simulink library "xpcnilib"  (Simulink 6.0)
settings: Solver=ode45  SolverMode=SingleTasking  StartTime=0.0  StopTime=10.0  RelTol=1e-3
undefined symbols (not defined in the file or in its folder): madnipcie, mctrnipcie, mctrnipciecap, mdacbisa, mdanipci670x, mdanipci671x, mdanipcie, mdionipci6527, mdionipcie, mencnipci660x, misa8255, mnigpib, mnipci660x, mpci8255
libraries: xpcmeasurementcomputinglib x6
(part 2 of 3)

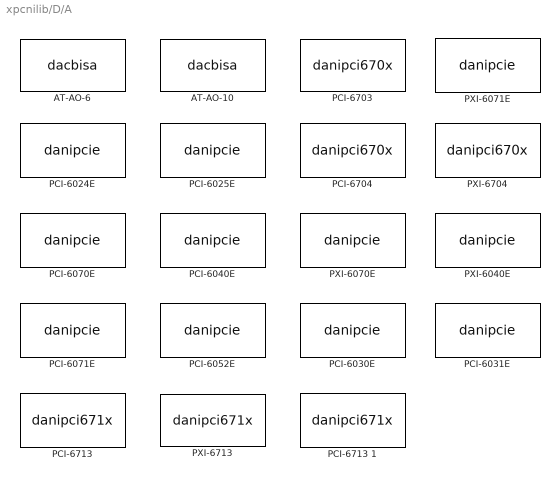
== system xpcnilib/D/A ==
  "AT-AO-10 " : S-Function  InitFcn=mdacbisa(1);  FunctionName=dacbisa  Parameters=channel, range, reset, initValue, sampletime, baseaddress, boardType  mask(dacbisa){channel=[1], range=[-10], reset=[1], initValue=[0], sampletime=0.001, baseaddress=0x300}
      mask prompts: channel "Channel vector:"; range "Range vector:"; reset "Reset vector:"; initValue "Initial value vector:"; sampletime "Sample time:"; baseaddress "Base address (i.e. 0xd000):"
      mask help:
      | AT-AO-10
      | National Instr.
      | Analog Output
      mask init:
      | baseaddress=hex2dec(baseaddress(3:end));
      | boardType=12;
      | [reset, initValue] = mdacbisa(2, channel, range, reset, initValue, baseaddress, boardType);
      mask Help: helpview(fullfile(docroot, 'mapfiles', 'xpc.map'), 'NationalInstruments_AT-AO-10_DA')
      mask Display: disp('AT-AO-10\nNational Instr.\nAnalog Output');port_label('input',1,'1');
  "AT-AO-6 " : S-Function  InitFcn=mdacbisa(1);  FunctionName=dacbisa  Parameters=channel, range, reset, initValue, sampletime, baseaddress, boardType  mask(dacbisa){channel=[1], range=[-10], reset=[1], initValue=[0], sampletime=0.001, baseaddress=0x300}
      mask prompts: channel "Channel vector:"; range "Range vector:"; reset "Reset vector:"; initValue "Initial value vector:"; sampletime "Sample time:"; baseaddress "Base address (i.e. 0xd000):"
      mask help:
      | AT-AO-6
      | National Instr.
      | Analog Output
      mask init:
      | baseaddress=hex2dec(baseaddress(3:end));
      | boardType=11;
      | [reset, initValue] = mdacbisa(2, channel, range, reset, initValue, baseaddress, boardType);
      mask Help: helpview(fullfile(docroot, 'mapfiles', 'xpc.map'), 'NationalInstruments_AT-AO-6_DA')
      mask Display: disp('AT-AO-6\nNational Instr.\nAnalog Output');port_label('input',1,'1');
  "PCI-6024E " : S-Function  InitFcn=mdanipcie(1);  FunctionName=danipcie  Parameters="channel, range, reset, initValue, sampletime, slot,  boardType"  mask(danipcie){channel=[1], reset=[1], initValue=[0], sampletime=0.001, slot=-1}
      mask prompts: channel "Channel vector:"; reset "Reset vector:"; initValue "Initial value vector:"; sampletime "Sample time:"; slot "PCI slot (-1: autosearch):"
      mask help:
      | PCI-6024E
      | National Instruments
      | Analog Output
      mask init:
      | boardType=2;
      | range=[];
      | [range,reset,initValue]=mdanipcie(2,channel, range, reset, initValue, slot, boardType);
      mask Help: helpview(fullfile(docroot, 'mapfiles', 'xpc.map'), 'NationalInstruments_PCI-6024E_DA')
      mask Display: disp('PCI-6024E\nNational Instr.\nAnalog Output');port_label('input',1,'1');
  "PCI-6025E " : S-Function  InitFcn=mdanipcie(1);  FunctionName=danipcie  Parameters="channel, range, reset, initValue, sampletime, slot,  boardType"  mask(danipcie){channel=[1], reset=[1], initValue=[0], sampletime=0.001, slot=-1}
      mask prompts: channel "Channel vector:"; reset "Reset vector:"; initValue "Initial value vector:"; sampletime "Sample time:"; slot "PCI slot (-1: autosearch):"
      mask help:
      | PCI-6025E
      | National Instruments
      | Analog Output
      mask init:
      | boardType=3;
      | range=[];
      | [range, reset, initValue]=mdanipcie(2,channel, range, reset, initValue, slot, boardType);
      mask Help: helpview(fullfile(docroot, 'mapfiles', 'xpc.map'), 'NationalInstruments_PCI-6025E_DA')
      mask Display: disp('PCI-6025E\nNational Instr.\nAnalog Output');port_label('input',1,'1');
  "PCI-6030E " : S-Function  InitFcn=mdanipcie(1);  FunctionName=danipcie  Parameters="channel, range, reset, initValue, sampletime, slot,  boardType"  mask(danipcie){channel=[1], range=[-10], reset=[1], initValue=[0], sampletime=0.001, slot=-1}
      mask prompts: channel "Channel vector:"; range "Range vector:"; reset "Reset vector:"; initValue "Initial value vector:"; sampletime "Sample time:"; slot "PCI slot (-1: autosearch):"
      mask help:
      | PCI-6030E
      | National Instruments
      | Analog Output
      mask init:
      | boardType=10;
      | [range,reset,initValue]=mdanipcie(2,channel, range, reset, initValue, slot, boardType);
      mask Help: helpview(fullfile(docroot, 'mapfiles', 'xpc.map'), 'NationalInstruments_PCI-MIO-16XE-10_DA')
      mask Display: disp('PCI-6030E\nNational Instr.\nAnalog Output');port_label('input',1,'1');
  "PCI-6031E " : S-Function  InitFcn=mdanipcie(1);  FunctionName=danipcie  Parameters="channel, range, reset, initValue, sampletime, slot,  boardType"  mask(danipcie){channel=[1], range=[-10], reset=[1], initValue=[0], sampletime=0.001, slot=-1}
      mask prompts: channel "Channel vector:"; range "Range vector:"; reset "Reset vector:"; initValue "Initial value vector:"; sampletime "Sample time:"; slot "PCI slot (-1: autosearch):"
      mask help:
      | PCI-6031E
      | National Instruments
      | Analog Output
      mask init:
      | boardType=11;
      | [range,reset,initValue]=mdanipcie(2,channel, range, reset, initValue, slot, boardType);
      mask Help: helpview(fullfile(docroot, 'mapfiles', 'xpc.map'), 'NationalInstruments_PCI-6031E_DA')
      mask Display: disp('PCI-6031E\nNational Instr.\nAnalog Output');port_label('input',1,'1');
  "PCI-6040E " : S-Function  InitFcn=mdanipcie(1);  FunctionName=danipcie  Parameters="channel, range, reset, initValue, sampletime, slot,  boardType"  mask(danipcie){channel=[1], range=[-10], reset=[1], initValue=[0], sampletime=0.001, slot=-1}
      mask prompts: channel "Channel vector:"; range "Range vector:"; reset "Reset vector:"; initValue "Initial value vector:"; sampletime "Sample time:"; slot "PCI slot (-1: autosearch):"
      mask help:
      | PCI-6040E
      | National Instruments
      | Analog Output
      mask init:
      | boardType=5;
      | [range,reset,initValue]=mdanipcie(2,channel, range, reset, initValue, slot, boardType);
      mask Help: helpview(fullfile(docroot, 'mapfiles', 'xpc.map'), 'NationalInstruments_PCI-MIO-16E-4_DA')
      mask Display: disp('PCI-6040E\nNational Instr.\nAnalog Output');port_label('input',1,'1');
  "PCI-6052E " : S-Function  InitFcn=mdanipcie(1);  FunctionName=danipcie  Parameters="channel, range, reset, initValue, sampletime, slot,  boardType"  mask(danipcie){channel=[1], range=[-10], reset=[1], initValue=[0], sampletime=0.001, slot=-1}
      mask prompts: channel "Channel vector:"; range "Range vector:"; reset "Reset vector:"; initValue "Initial value vector:"; sampletime "Sample time:"; slot "PCI slot (-1: autosearch):"
      mask help:
      | PCI-6052E
      | National Instruments
      | Analog Output
      mask init:
      | boardType=9;
      | [range,reset,initValue]=mdanipcie(2,channel, range, reset, initValue, slot, boardType);
      mask Help: helpview(fullfile(docroot, 'mapfiles', 'xpc.map'), 'NationalInstruments_PCI-6052E_DA')
      mask Display: disp('PCI-6052E\nNational Instr.\nAnalog Output');port_label('input',1,'1');
  "PCI-6070E " : S-Function  InitFcn=mdanipcie(1);  FunctionName=danipcie  Parameters="channel, range, reset, initValue, sampletime, slot,  boardType"  mask(danipcie){channel=[1], range=[-10], reset=[1], initValue=[0], sampletime=0.001, slot=-1}
      mask prompts: channel "Channel vector:"; range "Range vector:"; reset "Reset vector:"; initValue "Initial value vector:"; sampletime "Sample time:"; slot "PCI slot (-1: autosearch):"
      mask help:
      | PCI-6070E
      | National Instruments
      | Analog Output
      mask init:
      | boardType=4;
      | [range,reset,initValue]=mdanipcie(2,channel, range, reset, initValue, slot, boardType);
      mask Help: helpview(fullfile(docroot, 'mapfiles', 'xpc.map'), 'NationalInstruments_PCI-MIO-16E-1_DA')
      mask Display: disp('PCI-6070E\nNational Instr.\nAnalog Output');port_label('input',1,'1');
  "PCI-6071E " : S-Function  InitFcn=mdanipcie(1);  FunctionName=danipcie  Parameters="channel, range, reset, initValue, sampletime, slot,  boardType"  mask(danipcie){channel=[1], range=[-10], reset=[1], initValue=[0], sampletime=0.001, slot=-1}
      mask prompts: channel "Channel vector:"; range "Range vector:"; reset "Reset vector:"; initValue "Initial value vector:"; sampletime "Sample time:"; slot "PCI slot (-1: autosearch):"
      mask help:
      | PCI-6071E
      | National Instruments
      | Analog Output
      mask init:
      | boardType=8;
      | [range,reset,initValue]=mdanipcie(2,channel, range, reset, initValue, slot, boardType);
      mask Help: helpview(fullfile(docroot, 'mapfiles', 'xpc.map'), 'NationalInstruments_PCI-6071E_DA')
      mask Display: disp('PCI-6071E\nNational Instr.\nAnalog Output');port_label('input',1,'1');
  "PCI-6703 " : S-Function  InitFcn=mdanipci670x(1);  FunctionName=danipci670x  Parameters=channel, sampletime, pcislot, boardType  mask(danipci6703){channel=[1], sampletime=0.001, pcislot=-1}
      mask prompts: channel "Channel vector:"; sampletime "Sample time:"; pcislot "PCI slot (-1: autosearch):"
      mask help:
      | PCI-6703
      | National Instr.
      | Analog Output
      mask init:
      | boardType=1;
      | [maskdisplay, maskdescription]= mdanipci670x(2, boardType, channel, pcislot);
      | set_param(gcb,'MaskDescription',maskdescription);
      | set_param(gcb,'MaskDisplay',maskdisplay);
      mask Help: helpview(fullfile(docroot, 'mapfiles', 'xpc.map'), 'NationalInstruments_PCI-6703_DA')
      mask Display: disp('PCI-6703\nNational Instr.\nAnalog Output');port_label('input',1,'1');
  "PCI-6704 " : S-Function  InitFcn=mdanipci670x(1);  FunctionName=danipci670x  Parameters=channel, sampletime, pcislot, boardType  mask(danipci6704){channel=[1], sampletime=0.001, pcislot=-1}
      mask prompts: channel "Channel vector:"; sampletime "Sample time:"; pcislot "PCI slot (-1: autosearch):"
      mask help:
      | PCI-6704
      | National Instr.
      | Analog Output
      mask init:
      | boardType=2;
      | [maskdisplay, maskdescription]= mdanipci670x(2, boardType, channel, pcislot);
      | set_param(gcb,'MaskDescription',maskdescription);
      | set_param(gcb,'MaskDisplay',maskdisplay);
      mask Help: helpview(fullfile(docroot, 'mapfiles', 'xpc.map'), 'NationalInstruments_PCI-6704_DA')
      mask Display: disp('PCI-6704\nNational Instr.\nAnalog Output');port_label('input',1,'1');
  "PCI-6713 " : S-Function  InitFcn=mdanipci671x( 1, 1 );  FunctionName=danipci671x  Parameters=channel, sampletime, pcislot, boardType, reset, initval  mask(danipci6713){channel=[1], reset=[0], initval=[0], sampletime=0.001, pcislot=-1}
      mask prompts: channel "Channel vector:"; reset "Reset vector:"; initval "Initial value vector:"; sampletime "Sample time:"; pcislot "PCI slot (-1: autosearch):"
      mask help:
      | PCI-6713
      | National Instr.
      | Analog Output
      mask init:
      | boardType=1;
      | [maskdisplay, maskdescription, reset, initval]= mdanipci671x(2, boardType, channel, reset, initval, pcislot);
      | set_param(gcb,'MaskDescription',maskdescription);
      | set_param(gcb,'MaskDisplay',maskdisplay);
      mask Help: helpview(fullfile(docroot, 'mapfiles', 'xpc.map'), 'NationalInstruments_PCI-6713_DA')
      mask Display: disp('PCI-6713\nNational Instr.\nAnalog Output');port_label('input',1,'1');
  "PCI-6713 1 " : S-Function  InitFcn=mdanipci671x( 1, 1 );  FunctionName=danipci671x  Parameters=channel, sampletime, pcislot, boardType, reset, initval  mask(danipci6711){channel=[1], reset=[0], initval=[0], sampletime=0.001, pcislot=-1}
      mask prompts: channel "Channel vector:"; reset "Reset vector:"; initval "Initial value vector:"; sampletime "Sample time:"; pcislot "PCI slot (-1: autosearch):"
      mask help:
      | PCI-6711
      | National Instr.
      | Analog Output
      mask init:
      | boardType=3;
      | [maskdisplay, maskdescription, reset, initval]= mdanipci671x(2, boardType, channel, reset, initval, pcislot);
      | set_param(gcb,'MaskDescription',maskdescription);
      | set_param(gcb,'MaskDisplay',maskdisplay);
      mask Help: helpview(fullfile(docroot, 'mapfiles', 'xpc.map'), 'NationalInstruments_PCI-6711_DA')
      mask Display: disp('PCI-6711\nNational Instr.\nAnalog Output');port_label('input',1,'1');
  "PXI-6040E " : S-Function  InitFcn=mdanipcie(1);  FunctionName=danipcie  Parameters="channel, range, reset, initValue, sampletime, slot,  boardType"  mask(danipcie){channel=[1], range=[-10], reset=[1], initValue=[0], sampletime=0.001, slot=-1}
      mask prompts: channel "Channel vector:"; range "Range vector:"; reset "Reset vector:"; initValue "Initial value vector:"; sampletime "Sample time:"; slot "PCI slot (-1: autosearch):"
      mask help:
      | PXI-6040E
      | National Instruments
      | Analog Output
      mask init:
      | boardType=7;
      | [range,reset,initValue]=mdanipcie(2,channel, range, reset, initValue, slot, boardType);
      mask Help: helpview(fullfile(docroot, 'mapfiles', 'xpc.map'), 'NationalInstruments_PXI-6040E_DA')
      mask Display: disp('PXI-6040E\nNational Instr.\nAnalog Output');port_label('input',1,'1');
  "PXI-6070E " : S-Function  InitFcn=mdanipcie(1);  FunctionName=danipcie  Parameters="channel, range, reset, initValue, sampletime, slot,  boardType"  mask(danipcie){channel=[1], range=[-10], reset=[1], initValue=[0], sampletime=0.001, slot=-1}
      mask prompts: channel "Channel vector:"; range "Range vector:"; reset "Reset vector:"; initValue "Initial value vector:"; sampletime "Sample time:"; slot "PCI slot (-1: autosearch):"
      mask help:
      | PXI-6070E
      | National Instruments
      | Analog Output
      mask init:
      | boardType=6;
      | [range,reset,initValue]=mdanipcie(2,channel, range, reset, initValue, slot, boardType);
      mask Help: helpview(fullfile(docroot, 'mapfiles', 'xpc.map'), 'NationalInstruments_PXI-6070E_DA')
      mask Display: disp('PXI-6070E\nNational Instr.\nAnalog Output');port_label('input',1,'1');
  "PXI-6071E " : S-Function  InitFcn=mdanipcie(1);  FunctionName=danipcie  Parameters="channel, range, reset, initValue, sampletime, slot,  boardType"  mask(danipcie){channel=[1], range=[-10], reset=[1], initValue=[0], sampletime=0.001, slot=-1}
      mask prompts: channel "Channel vector:"; range "Range vector:"; reset "Reset vector:"; initValue "Initial value vector:"; sampletime "Sample time:"; slot "PCI slot (-1: autosearch):"
      mask help:
      | PXI-6071E
      | National Instruments
      | Analog Output
      mask init:
      | boardType=12;
      | [range,reset,initValue]=mdanipcie(2,channel, range, reset, initValue, slot, boardType);
      mask Help: helpview(fullfile(docroot, 'mapfiles', 'xpc.map'), 'NationalInstruments_PXI-6071E_DA')
      mask Display: disp('PXI-6071E\nNational Instr.\nAnalog Output');port_label('input',1,'1');
  "PXI-6704 " : S-Function  InitFcn=mdanipci670x(1);  FunctionName=danipci670x  Parameters=channel, sampletime, pcislot, boardType  mask(danipxi6704){channel=[1], sampletime=0.001, pcislot=-1}
      mask prompts: channel "Channel vector:"; sampletime "Sample time:"; pcislot "PCI slot (-1: autosearch):"
      mask help:
      | PXI-6704
      | National Instr.
      | Analog Output
      mask init:
      | boardType=3;
      | [maskdisplay, maskdescription]= mdanipci670x(2, boardType, channel, pcislot);
      | set_param(gcb,'MaskDescription',maskdescription);
      | set_param(gcb,'MaskDisplay',maskdisplay);
      mask Help: helpview(fullfile(docroot, 'mapfiles', 'xpc.map'), 'NationalInstruments_PCI-6704_DA')
      mask Display: disp('PXI-6704\nNational Instr.\nAnalog Output');port_label('input',1,'1');
  "PXI-6713 " : S-Function  InitFcn=mdanipci671x( 1, 2 );  FunctionName=danipci671x  Parameters=channel, sampletime, pcislot, boardType, reset, initval  mask(danipxi6713){channel=[1], reset=[0], initval=[0], sampletime=0.001, pcislot=-1}
      mask prompts: channel "Channel vector:"; reset "Reset vector:"; initval "Initial value vector:"; sampletime "Sample time:"; pcislot "PCI slot (-1: autosearch):"
      mask help:
      | PXI-6713
      | National Instr.
      | Analog Output
      mask init:
      | boardType=2;
      | [maskdisplay, maskdescription, reset, initval]= mdanipci671x(2, boardType, channel, reset, initval, pcislot);
      | set_param(gcb,'MaskDescription',maskdescription);
      | set_param(gcb,'MaskDisplay',maskdisplay);
      mask Help: helpview(fullfile(docroot, 'mapfiles', 'xpc.map'), 'NationalInstruments_PXI-6713_DA')
      mask Display: disp('PXI-6713\nNational Instr.\nAnalog Output');port_label('input',1,'1');

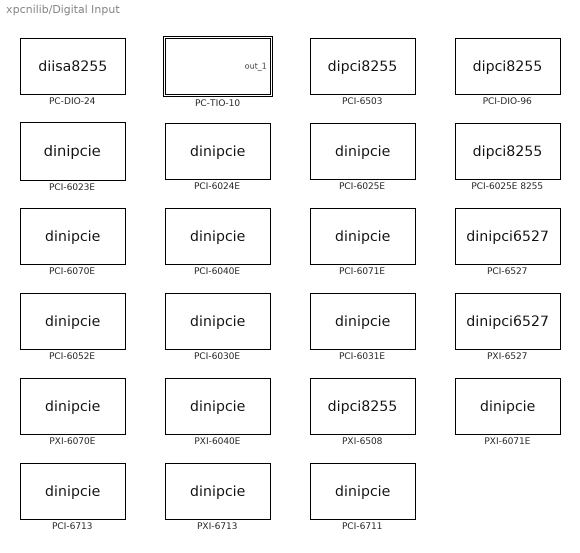
== system xpcnilib/Digital Input ==
  "PC-DIO-24 " : S-Function  InitFcn=misa8255(1);  FunctionName=diisa8255  Parameters=channel, port, sampletime, baseaddress, control  mask(dinipcdio24){channel=[1], port=A, chip=1, sampletime=0.001, baseaddress=0x300}
      mask prompts: channel "Channel vector:"; sampletime "Sample time:"; baseaddress "Base address (i.e. 0xd000):"
      mask help:
      | PC-DIO-24
      | National Instruments
      | Digital Input
      mask init:
      | baseaddress=hex2dec(baseaddress(3:end));
      | control=155;
      | boardType=16;
      | [baseaddress,control,maskdisplay,maskdescription]=misa8255(2, chip, port, channel, baseaddress);
      | set_param(gcb, 'MaskDisplay', maskdisplay);
      | set_param(gcb, 'MaskDescription', maskdescription);
      mask Help: helpview(fullfile(docroot, 'mapfiles', 'xpc.map'), 'NationalInstruments_PC-DIO-24_DIN')
      mask StyleString: edit,popup(A|B|C),popup(1),edit,edit
      mask Display: disp('PC-DIO-24\nNational Instr.\nDigital Input');port_label('output',1,'1');
  "PC-TIO-10 " : Subsystem  PropExecContextAcrossSSBoundary=on  mask(Digital Input Module){n_channels=1, port=PIA A, sample_time=0.001, baseaddress=0x300}
      mask prompts: n_channels "Number of channels:"; sample_time "Sample time:"; baseaddress "Base address (i.e. 0xd000):"
      mask help:
      | PC-TIO-10
      | National Instruments
      | Digital Input
      mask init:
      | baseaddress=hex2dec(baseaddress(3:end));
      mask Help: helpview(fullfile(docroot, 'mapfiles', 'xpc.map'), 'NationalInstruments_PC-TIO-10_DIN')
      mask StyleString: edit,popup(PIA A|PIA B),edit,edit
      mask Display: disp('PC-TIO-10\nNational Instr.\nDigital Input')
  "PCI-6023E " : S-Function  InitFcn=mdionipcie(1);  FunctionName=dinipcie  Parameters=channel,sampletime,slot, control, boardType  mask(donipcie){channel=[1], sampletime=0.001, slot=-1}
      mask prompts: channel "Channel vector:"; sampletime "Sample time:"; slot "PCI slot (-1: autosearch):"
      mask help:
      | PCI-6023E
      | National Instruments
      | Digital Input
      mask init:
      | control=0;
      | boardType=1;
      | control=mdionipcie(2,channel,slot,1,boardType);
      mask Help: helpview(fullfile(docroot, 'mapfiles', 'xpc.map'), 'NationalInstruments_PCI-6023E_DIN')
      mask Display: disp('PCI-6023E\nNational Instr.\nDigital Input');port_label('output',1,'1');
  "PCI-6024E " : S-Function  InitFcn=mdionipcie(1);  FunctionName=dinipcie  Parameters=channel,sampletime,slot, control, boardType  mask(donipcie){channel=[1], sampletime=0.001, slot=-1}
      mask prompts: channel "Channel vector:"; sampletime "Sample time:"; slot "PCI slot (-1: autosearch):"
      mask help:
      | PCI-6024E
      | National Instruments
      | Digital Input
      mask init:
      | control=0;
      | boardType=2;
      | control=mdionipcie(2,channel,slot,1,boardType);
      mask Help: helpview(fullfile(docroot, 'mapfiles', 'xpc.map'), 'NationalInstruments_PCI-6024E_DIN')
      mask Display: disp('PCI-6024E\nNational Instr.\nDigital Input');port_label('output',1,'1');
  "PCI-6025E " : S-Function  InitFcn=mdionipcie(1);  FunctionName=dinipcie  Parameters=channel,sampletime,slot, control, boardType  mask(donipcie){channel=[1], sampletime=0.001, slot=-1}
      mask prompts: channel "Channel vector:"; sampletime "Sample time:"; slot "PCI slot (-1: autosearch):"
      mask help:
      | PCI-6025E
      | National Instruments
      | Digital Input
      mask init:
      | control=0;
      | boardType=3;
      | control=mdionipcie(2,channel,slot,1,boardType);
      mask Help: helpview(fullfile(docroot, 'mapfiles', 'xpc.map'), 'NationalInstruments_PCI-6025E_DIN')
      mask Display: disp('PCI-6025E\nNational Instr.\nDigital Input');port_label('output',1,'1');
  "PCI-6025E 8255 " : S-Function  InitFcn=mpci8255(1);  FunctionName=dipci8255  Parameters=channel, port, chip, sampletime, slot, control, boardType  mask(dinipci6025e8255){channel=[1], port=A, chip=1, sampletime=0.001, slot=-1}
      mask prompts: channel "Channel vector:"; sampletime "Sample time:"; slot "PCI slot (-1: autosearch):"
      mask help:
      | PCI-6025E (8255)
      | National Instruments
      | Digital Input
      mask init:
      | control=155;
      | [boardType,control,maskdisplay,maskdescription]=mpci8255(2, chip, port, channel, slot);
      | set_param(gcb, 'MaskDisplay', maskdisplay);
      | set_param(gcb, 'MaskDescription', maskdescription);
      mask Help: helpview(fullfile(docroot, 'mapfiles', 'xpc.map'), 'NationalInstruments_PCI-6025E-8255_DIN')
      mask StyleString: edit,popup(A|B|C),popup(1),edit,edit
      mask Display: disp('PCI-6025E (8255)\nNational Instr.\nDigital Input');port_label('output',1,'1');
  "PCI-6030E " : S-Function  InitFcn=mdionipcie(1);  FunctionName=dinipcie  Parameters=channel,sampletime,slot, control, boardType  mask(donipcie){channel=[1], sampletime=0.001, slot=-1}
      mask prompts: channel "Channel vector:"; sampletime "Sample time:"; slot "PCI slot (-1: autosearch):"
      mask help:
      | PCI-6030E
      | National Instruments
      | Digital Input
      mask init:
      | control=0;
      | boardType=10;
      | control=mdionipcie(2,channel,slot,1,boardType);
      mask Help: helpview(fullfile(docroot, 'mapfiles', 'xpc.map'), 'NationalInstruments_PCI-MIO-16XE-10_DIN')
      mask Display: disp('PCI-6030E\nNational Instr.\nDigital Input');port_label('output',1,'1');
  "PCI-6031E " : S-Function  InitFcn=mdionipcie(1);  FunctionName=dinipcie  Parameters=channel,sampletime,slot, control, boardType  mask(donipcie){channel=[1], sampletime=0.001, slot=-1}
      mask prompts: channel "Channel vector:"; sampletime "Sample time:"; slot "PCI slot (-1: autosearch):"
      mask help:
      | PCI-6031E
      | National Instruments
      | Digital Input
      mask init:
      | control=0;
      | boardType=11;
      | control=mdionipcie(2,channel,slot,1,boardType);
      mask Help: helpview(fullfile(docroot, 'mapfiles', 'xpc.map'), 'NationalInstruments_PCI-6031E_DIN')
      mask Display: disp('PCI-6031E\nNational Instr.\nDigital Input');port_label('output',1,'1');
  "PCI-6040E " : S-Function  InitFcn=mdionipcie(1);  FunctionName=dinipcie  Parameters=channel,sampletime,slot, control, boardType  mask(donipcie){channel=[1], sampletime=0.001, slot=-1}
      mask prompts: channel "Channel vector:"; sampletime "Sample time:"; slot "PCI slot (-1: autosearch):"
      mask help:
      | PCI-6040E
      | National Instruments
      | Digital Input
      mask init:
      | control=0;
      | boardType=5;
      | control=mdionipcie(2,channel,slot,1,boardType);
      mask Help: helpview(fullfile(docroot, 'mapfiles', 'xpc.map'), 'NationalInstruments_PCI-MIO-16E-4_DIN')
      mask Display: disp('PCI-6040E\nNational Instr.\nDigital Input');port_label('output',1,'1');
  "PCI-6052E " : S-Function  InitFcn=mdionipcie(1);  FunctionName=dinipcie  Parameters=channel,sampletime,slot, control, boardType  mask(donipcie){channel=[1], sampletime=0.001, slot=-1}
      mask prompts: channel "Channel vector:"; sampletime "Sample time:"; slot "PCI slot (-1: autosearch):"
      mask help:
      | PCI-6052E
      | National Instruments
      | Digital Input
      mask init:
      | control=0;
      | boardType=9;
      | control=mdionipcie(2,channel,slot,1,boardType);
      mask Help: helpview(fullfile(docroot, 'mapfiles', 'xpc.map'), 'NationalInstruments_PCI-6052E_DIN')
      mask Display: disp('PCI-6052E\nNational Instr.\nDigital Input');port_label('output',1,'1');
  "PCI-6070E " : S-Function  InitFcn=mdionipcie(1);  FunctionName=dinipcie  Parameters=channel,sampletime,slot, control, boardType  mask(donipcie){channel=[1], sampletime=0.001, slot=-1}
      mask prompts: channel "Channel vector:"; sampletime "Sample time:"; slot "PCI slot (-1: autosearch):"
      mask help:
      | PCI-6070E
      | National Instruments
      | Digital Input
      mask init:
      | control=0;
      | boardType=4;
      | control=mdionipcie(2,channel,slot,1,boardType);
      mask Help: helpview(fullfile(docroot, 'mapfiles', 'xpc.map'), 'NationalInstruments_PCI-MIO-16E-1_DIN')
      mask Display: disp('PCI-6070E\nNational Instr.\nDigital Input');port_label('output',1,'1');
  "PCI-6071E " : S-Function  InitFcn=mdionipcie(1);  FunctionName=dinipcie  Parameters=channel,sampletime,slot, control, boardType  mask(donipcie){channel=[1], sampletime=0.001, slot=-1}
      mask prompts: channel "Channel vector:"; sampletime "Sample time:"; slot "PCI slot (-1: autosearch):"
      mask help:
      | PCI-6071E
      | National Instruments
      | Digital Input
      mask init:
      | control=0;
      | boardType=8;
      | control=mdionipcie(2,channel,slot,1,boardType);
      mask Help: helpview(fullfile(docroot, 'mapfiles', 'xpc.map'), 'NationalInstruments_PCI-6071E_DIN')
      mask Display: disp('PCI-6071E\nNational Instr.\nDigital Input');port_label('output',1,'1');
  "PCI-6503 " : S-Function  InitFcn=mpci8255(1);  FunctionName=dipci8255  Parameters=channel, port, chip, sampletime, slot, control, boardType  mask(dinipci6503){channel=[1], port=A, chip=1, sampletime=0.001, slot=-1}
      mask prompts: channel "Channel vector:"; sampletime "Sample time:"; slot "PCI slot (-1: autosearch):"
      mask help:
      | PCI-6503
      | National Instruments
      | Digital Input
      mask init:
      | control=155;
      | [boardType,control,maskdisplay,maskdescription]=mpci8255(2, chip, port, channel, slot);
      | set_param(gcb, 'MaskDisplay', maskdisplay);
      | set_param(gcb, 'MaskDescription', maskdescription);
      mask Help: helpview(fullfile(docroot, 'mapfiles', 'xpc.map'), 'NationalInstruments_PCI-6503_DIN')
      mask StyleString: edit,popup(A|B|C),popup(1),edit,edit
      mask Display: disp('PCI-6503\nNational Instr.\nDigital Input');port_label('output',1,'1');
  "PCI-6527 " : S-Function  InitFcn=mdionipci6527(1);  FunctionName=dinipci6527  Parameters=channel, port, sample, slot, filter, filtertime,1  mask(dinipci6527){channel=[1], port=A, filter=[0], filtertime=0, sample=.001, slot=-1}
      mask prompts: channel "Channel vector:"; filter "Filter vector:"; filtertime "Filter interval:"; sample "Sample time:"; slot "PCI slot (-1: autosearch):"
      mask help:
      | PCI-6527
      | National Instruments
      | Digital Input
      mask init:
      | filter = mdionipci6527( 2, channel, port, sample, slot, 1, filter, filtertime, 0, 0 );
      mask Help: helpview(fullfile(docroot, 'mapfiles', 'xpc.map'), 'NationalInstruments_PCI-6527_DIN')
      mask StyleString: edit,popup(A|B|C),edit,edit,edit,edit
      mask Display: disp('PCI-6527\nNational Instr\nDigital Input');port_label('output',1,'1');
  "PCI-6711 " : S-Function  InitFcn=mdionipcie(1);  FunctionName=dinipcie  Parameters=channel,sampletime,slot, control, boardType  mask(donipcie){channel=[1], sampletime=0.001, slot=-1}
      mask prompts: channel "Channel vector:"; sampletime "Sample time:"; slot "PCI slot (-1: autosearch):"
      mask help:
      | PCI-6711
      | National Instruments
      | Digital Input
      mask init:
      | control=0;
      | boardType=15;
      | control=mdionipcie(2,channel,slot,1,boardType);
      mask Help: helpview(fullfile(docroot, 'mapfiles', 'xpc.map'), 'NationalInstruments_PCI-6711_DIN')
      mask Display: disp('PCI-6711 \nNational Instr.\nDigital Input');port_label('output',1,'1');
  "PCI-6713 " : S-Function  InitFcn=mdionipcie(1);  FunctionName=dinipcie  Parameters=channel,sampletime,slot, control, boardType  mask(donipcie){channel=[1], sampletime=0.001, slot=-1}
      mask prompts: channel "Channel vector:"; sampletime "Sample time:"; slot "PCI slot (-1: autosearch):"
      mask help:
      | PCI-6713
      | National Instruments
      | Digital Input
      mask init:
      | control=0;
      | boardType=13;
      | control=mdionipcie(2,channel,slot,1,boardType);
      mask Help: helpview(fullfile(docroot, 'mapfiles', 'xpc.map'), 'NationalInstruments_PCI-6713_DIN')
      mask Display: disp('PCI-6713 \nNational Instr.\nDigital Input');port_label('output',1,'1');
  "PCI-DIO-96 " : S-Function  InitFcn=mpci8255(1);  FunctionName=dipci8255  Parameters=channel, port, chip, sampletime, slot, control, boardType  mask(dinipcidio96){channel=[1], port=A, chip=1, sampletime=0.001, slot=-1}
      mask prompts: channel "Channel vector:"; sampletime "Sample time:"; slot "PCI slot (-1: autosearch):"
      mask help:
      | PCI-DIO-96
      | National Instruments
      | Digital Input
      mask init:
      | control=155;
      | [boardType,control,maskdisplay,maskdescription]=mpci8255(2, chip, port, channel, slot);
      | set_param(gcb, 'MaskDisplay', maskdisplay);
      | set_param(gcb, 'MaskDescription', maskdescription);
      mask Help: helpview(fullfile(docroot, 'mapfiles', 'xpc.map'), 'NationalInstruments_PCI-DIO-96_DIN')
      mask StyleString: edit,popup(A|B|C),popup(1|2|3|4),edit,edit
      mask Display: disp('PCI-DIO-96\nNational Instr.\nDigital Input');port_label('output',1,'1');
  "PXI-6040E " : S-Function  InitFcn=mdionipcie(1);  FunctionName=dinipcie  Parameters=channel,sampletime,slot, control, boardType  mask(donipcie){channel=[1], sampletime=0.001, slot=-1}
      mask prompts: channel "Channel vector:"; sampletime "Sample time:"; slot "PCI slot (-1: autosearch):"
      mask help:
      | PXI-6040E
      | National Instruments
      | Digital Input
      mask init:
      | control=0;
      | boardType=7;
      | control=mdionipcie(2,channel,slot,1,boardType);
      mask Help: helpview(fullfile(docroot, 'mapfiles', 'xpc.map'), 'NationalInstruments_PXI-6040E_DIN')
      mask Display: disp('PXI-6040E\nNational Instr.\nDigital Input');port_label('output',1,'1');
  "PXI-6070E " : S-Function  InitFcn=mdionipcie(1);  FunctionName=dinipcie  Parameters=channel,sampletime,slot, control, boardType  mask(donipcie){channel=[1], sampletime=0.001, slot=-1}
      mask prompts: channel "Channel vector:"; sampletime "Sample time:"; slot "PCI slot (-1: autosearch):"
      mask help:
      | PXI-6070E
      | National Instruments
      | Digital Input
      mask init:
      | control=0;
      | boardType=6;
      | control=mdionipcie(2,channel,slot,1,boardType);
      mask Help: helpview(fullfile(docroot, 'mapfiles', 'xpc.map'), 'NationalInstruments_PXI-6070E_DIN')
      mask Display: disp('PXI-6070E\nNational Instr.\nDigital Input');port_label('output',1,'1');
  "PXI-6071E " : S-Function  InitFcn=mdionipcie(1);  FunctionName=dinipcie  Parameters=channel,sampletime,slot, control, boardType  mask(donipcie){channel=[1], sampletime=0.001, slot=-1}
      mask prompts: channel "Channel vector:"; sampletime "Sample time:"; slot "PCI slot (-1: autosearch):"
      mask help:
      | PXI-6071E
      | National Instruments
      | Digital Input
      mask init:
      | control=0;
      | boardType=12;
      | control=mdionipcie(2,channel,slot,1,boardType);
      mask Help: helpview(fullfile(docroot, 'mapfiles', 'xpc.map'), 'NationalInstruments_PXI-6071E_DIN')
      mask Display: disp('PXI-6071E\nNational Instr.\nDigital Input');port_label('output',1,'1');
  "PXI-6508 " : S-Function  InitFcn=mpci8255(1);  FunctionName=dipci8255  Parameters=channel, port, chip, sampletime, slot, control, boardType  mask(dinipxi6508){channel=[1], port=A, chip=1, sampletime=0.001, slot=-1}
      mask prompts: channel "Channel vector:"; sampletime "Sample time:"; slot "PCI slot (-1: autosearch):"
      mask help:
      | PXI-6508
      | National Instruments
      | Digital Input
      mask init:
      | control=155;
      | [boardType,control,maskdisplay,maskdescription]=mpci8255(2, chip, port, channel, slot);
      | set_param(gcb, 'MaskDisplay', maskdisplay);
      | set_param(gcb, 'MaskDescription', maskdescription);
      mask Help: helpview(fullfile(docroot, 'mapfiles', 'xpc.map'), 'NationalInstruments_PXI-6508_DIN')
      mask StyleString: edit,popup(A|B|C),popup(1|2|3|4),edit,edit
      mask Display: disp('PXI-6508\nNational Instr.\nDigital Input');port_label('output',1,'1');
  "PXI-6527 " : S-Function  InitFcn=mdionipci6527(1);  FunctionName=dinipci6527  Parameters=channel, port, sample, slot, filter, filtertime,2  mask(dinipxi6527){channel=[1], port=A, filter=[0], filtertime=0, sample=.001, slot=-1}
      mask prompts: channel "Channel vector:"; filter "Filter vector:"; filtertime "Filter interval:"; sample "Sample time:"; slot "PCI slot (-1: autosearch):"
      mask help:
      | PXI-6527
      | National Instruments
      | Digital Input
      mask init:
      | filter = mdionipci6527( 2, channel, port, sample, slot, 1, filter, filtertime );
      mask Help: helpview(fullfile(docroot, 'mapfiles', 'xpc.map'), 'NationalInstruments_PXI-6527_DIN')
      mask StyleString: edit,popup(A|B|C),edit,edit,edit,edit
      mask Display: disp('PXI-6527\nNational Instr\nDigital Input');port_label('output',1,'1');
  "PXI-6713 " : S-Function  InitFcn=mdionipcie(1);  FunctionName=dinipcie  Parameters=channel,sampletime,slot, control, boardType  mask(donipcie){channel=[1], sampletime=0.001, slot=-1}
      mask prompts: channel "Channel vector:"; sampletime "Sample time:"; slot "PCI slot (-1: autosearch):"
      mask help:
      | PXI-6713
      | National Instruments
      | Digital Input
      mask init:
      | control=0;
      | boardType=14;
      | control=mdionipcie(2,channel,slot,1,boardType);
      mask Help: helpview(fullfile(docroot, 'mapfiles', 'xpc.map'), 'NationalInstruments_PXI-6713_DIN')
      mask Display: disp('PXI-6713 \nNational Instr.\nDigital Input');port_label('output',1,'1');
